simulink model "PTC_MBDS_DeadBand_Sample"  (R2013a)
settings: Solver=FixedStepDiscrete  StartTime=0.0  StopTime=100  FixedStep=Auto  RelTol=1e-3
undefined symbols (not defined in the file): sigbuilder_block
libraries: simulink_extras x1, PTC_MBDS_LIB x1
settings Model: Creator=uidl7367  LastModifiedBy=sundeep.tuteja
settings DataIOCC: SignalLoggingSaveFormat=ModelDataLogs
settings OptimizationCC: ExpressionDepthLimit=2147483647  InitFltsAndDblsToZero=on
settings DebuggingCC: SaveWithParameterizedLinksMsg=none  SignalResolutionControl=TryResolveAllWithWarning  SolverPrmCheckMsg=none  InheritedTsInSrcMsg=none  MultiTaskDSMMsg=warning  MultiTaskCondExecSysMsg=none  FcnCallInpInsideContextMsg=UseLocalSettings  StrictBusMsg=Warning
settings RTWCC: IncludeERTFirstTime=on
settings GRTTargetCC: TargetFcnLib=ansi_tfl_tmw.mat  CombineOutputUpdateFcns=off  GRTInterface=on

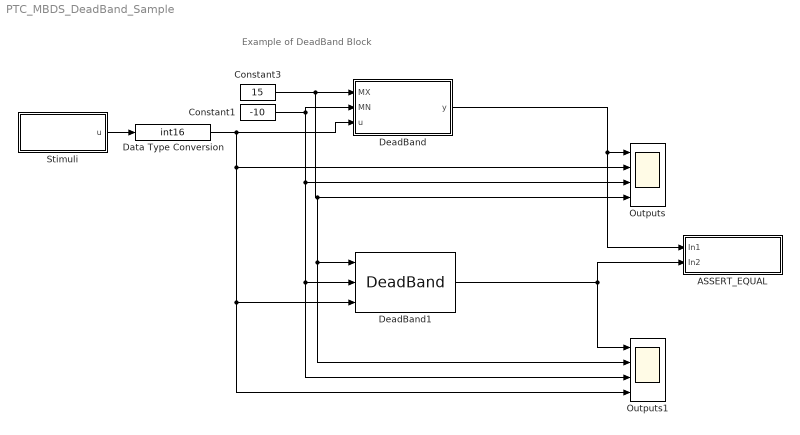
== system PTC_MBDS_DeadBand_Sample ==
  note: Example of DeadBand Block
  ASSERT_EQUAL : Subsystem
  Constant1 : Constant  InitFcn=|  Value=-10  VectorParams1D=off  OutDataTypeStr=Inherit: Inherit via back propagation
      | if(exist('MBDS_BlockCallback', 'file'))
      |    MBDS_BlockCallback('Update', gcb);  
      | end
  Constant3 : Constant  InitFcn=|  Value=15  VectorParams1D=off  OutDataTypeStr=Inherit: Inherit via back propagation
      | if(exist('MBDS_BlockCallback', 'file'))
      |    MBDS_BlockCallback('Update', gcb);  
      | end
  Data Type Conversion : DataTypeConversion  InitFcn=|  OutDataTypeStr=int16  SaturateOnIntegerOverflow=on
      | try
      |    MBDS_BlockCallback('Update', gcb);
      | end
  DeadBand : Subsystem  InitFcn=|  mask(DeadBand){MBDS_LibraryBlock=on, MBDS_BlockVersion=05.40}
      | if(exist('MBDS_BlockCallback', 'file'))
      |    MBDS_BlockCallback('Update', gcb);
      | end
      mask prompts: MBDS_LibraryBlock "MBDS library block"; MBDS_BlockVersion "Block version:"
      mask help: Returns zero, if the input value is between minimum (MN) and maximum (MX). Otherwise the output signal equals to the input signal reduced by the limits.
      mask init:
      | if(exist('MBDS_BlockCallback', 'file'))
      |    MBDS_BlockCallback('Init', gcb);
      | else
      |    % Disable all mask parameters
      |    MaskEnables = get_param(gcb, 'MaskEnables');
      |    for k = [1:length(MaskEnables)]
      |       MaskEnables{k} = 'off';
      |    end
      |    if(~isequal(MaskEnables, get_param(gcb, 'MaskEnables')))
      |       set_param(gcb, 'MaskEnables', MaskEnables);
      |    end
      | end
      mask Help: eval(['open([workdir(''library_dir:''),''\Blockset\help\'',get_param(gcb,''MaskType''),''.html''])'])
      mask Display:
      | % Show icon or block text
      | if(exist('DeadBand.tif', 'file'))
      |    image(imread('DeadBand.tif','tif'), [0.295739348370927 0.17 0.378947368421053 0.66]);
      |    disp('')
      | else
      |    disp(sprintf('Dead\nBand'));
      | end
      | 
      | % Display port labels
      | port_label('input', 1, 'MX');
      | port_label('input', 2, 'MN');
      | port_label('input', 3, 'u');
      | port_label('output', 1, 'y');
  DeadBand1 : PTC_MBDS_LIB/MBDS Standard Library/Basic Operations/Non-Linear Operations/DeadBand  PTC_MBDS_BlockVersion=5.32  PTC_BlockType=PTC_MBDS_DeadBand
  Outputs : Scope  NumInputPorts=4
      settings: TimeRange=10  YMin=-10~-20~-11~14  YMax=0~-10~-9~16  SampleInput=on  SampleTime=1
  Outputs1 : Scope  NumInputPorts=4
      settings: TimeRange=10  YMin=-10~-20~-11~14  YMax=0~-10~-9~16  SampleInput=on  SampleTime=1
  Stimuli : Subsystem  Tag=STV Subsys  LoadFcn=sigbuilder_block('load');  StartFcn=sigbuilder_block('start');  StopFcn=sigbuilder_block('stop');  ClipboardFcn=sigbuilder_block('clipboard');  mask(Sigbuilder block){}
      mask help: Sigbuilder GUI
      mask init:
      | if ~strcmp(get_param(bdroot(gcb),'SimulationStatus'),'stopped') tuvar = sigbuilder_block('maskInit'); end
      settings: CopyFcn=sigbuilder_block('copy');  DeleteFcn=sigbuilder_block('delete');  ModelCloseFcn=sigbuilder_block('modelClose');  PreSaveFcn=sigbuilder_block('preSave');  PauseFcn=sigbuilder_block('pause')  ContinueFcn=sigbuilder_block('continue')  NameChangeFcn=sigbuilder_block('namechange');  OpenFcn=sigbuilder_block('open',[45 129.75 470.25 423.75 ]);  CloseFcn=sigbuilder_block('close');
      mask Display: plot(0,0,100,100,[10,10,40,40,10],[80,20,20,80,80],[40,10],[50,50], [40,27,10],[65,72,56],[40,25,25,10],[28,28,43,43]);
  wires:
  Stimuli/1(u) -> Data Type Conversion/1
  DeadBand/1(y) -> ASSERT_EQUAL/1(In1), Outputs/1
  Constant3/1 -> DeadBand/1(MX), DeadBand1/1, Outputs1/2, Outputs/4
  Constant1/1 -> DeadBand/2(MN), DeadBand1/2, Outputs1/3, Outputs/3
  Data Type Conversion/1 -> DeadBand/3(u), DeadBand1/3, Outputs1/4, Outputs/2
  DeadBand1/1 -> ASSERT_EQUAL/2(In2), Outputs1/1

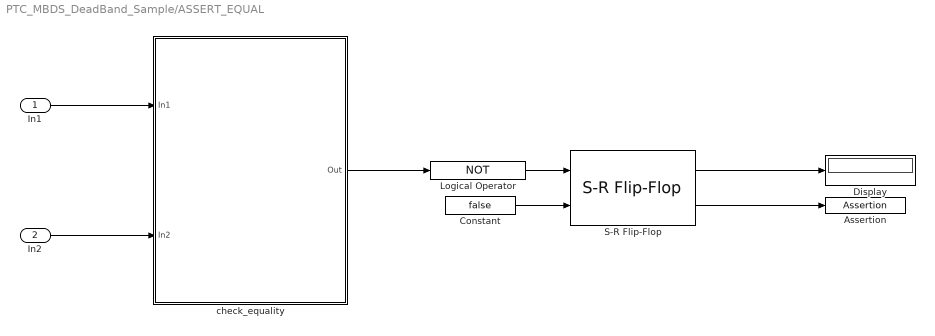
== system PTC_MBDS_DeadBand_Sample/ASSERT_EQUAL ==
  In1 : Inport
  In2 : Inport  Port=2
  Assertion : Assertion
  Constant : Constant  Value=false
  Display : Display
  Logical Operator : Logic  Operator=NOT  AllPortsSameDT=off  OutDataTypeStr=boolean
  S-R Flip-Flop : simulink_extras/Flip Flops/S-R Flip-Flop  initial_condition=0
  check_equality : MATLAB Function  TreatAsAtomicUnit=on
  wires:
  S-R Flip-Flop/1 -> Display/1
  check_equality/1(Out) -> Logical Operator/1
  Constant/1 -> S-R Flip-Flop/2
  S-R Flip-Flop/2 -> Assertion/1
  In2/1 -> check_equality/2(In2)
  In1/1 -> check_equality/1(In1)
  Logical Operator/1 -> S-R Flip-Flop/1

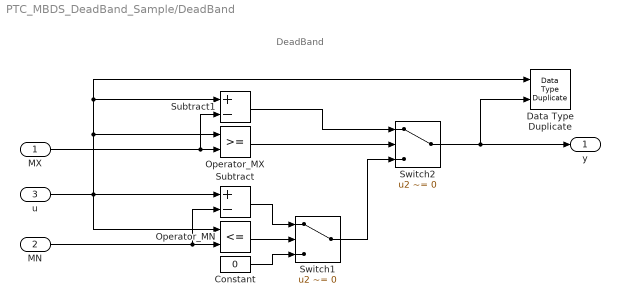
== system PTC_MBDS_DeadBand_Sample/DeadBand ==
  note: DeadBand
  MX : Inport
  MN : Inport  Port=2
  u : Inport  Port=3
  Constant : Constant  Value=0  OutDataTypeStr=Inherit: Inherit via back propagation
  Data Type Duplicate : DataTypeDuplicate
  Operator_MN : RelationalOperator  Operator=<=  OutDataTypeStr=boolean
  Operator_MX : RelationalOperator  OutDataTypeStr=boolean
  Subtract : Sum  Inputs=+-  OutDataTypeStr=Inherit: Inherit via back propagation  SaturateOnIntegerOverflow=on
  Subtract1 : Sum  Inputs=+-  OutDataTypeStr=Inherit: Inherit via back propagation  SaturateOnIntegerOverflow=on
  Switch1 : Switch  Criteria=u2 ~= 0  OutDataTypeStr=Inherit: Inherit via back propagation  SaturateOnIntegerOverflow=on
  Switch2 : Switch  Criteria=u2 ~= 0  OutDataTypeStr=Inherit: Inherit via back propagation  SaturateOnIntegerOverflow=on
  y : Outport
  wires:
  Subtract1/1 -> Switch2/1
  u/1 -> Operator_MX/1, Data Type Duplicate/1, Subtract1/1, Operator_MN/1, Subtract/1
  Constant/1 -> Switch1/3
  Subtract/1 -> Switch1/1
  MN/1 -> Operator_MN/2, Subtract/2
  Switch1/1 -> Switch2/3
  MX/1 -> Operator_MX/2, Subtract1/2
  Operator_MX/1 -> Switch2/2
  Operator_MN/1 -> Switch1/2
  Switch2/1 -> y/1, Data Type Duplicate/2

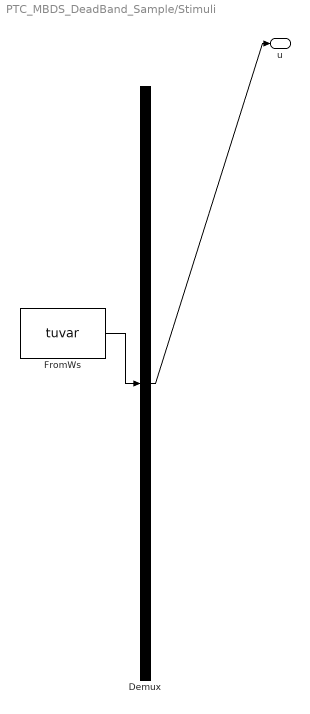
== system PTC_MBDS_DeadBand_Sample/Stimuli ==
  Demux : Demux  Tag=STV Demux  Outputs=1
  FromWs : FromWorkspace  Tag=STV FromWs  VariableName=tuvar  SampleTime=1  OutputAfterFinalValue=Holding final value
      SigBuilderData=|
      | common.afterFinalStr = 'Hold final value'
      | common.sampleTime = 1
      | dataSet.timeRange = [0 10]
      | dataSet.name = 'test data'
      | sbobj.Groups.Name = 'test data'
      | sbobj.Groups.Signals.Name = 'u'
      | sbobj.Groups.Signals.XData = [0 2 4 6 8 10]
      | sbobj.Groups.Signals.YData = [-20 -18 -16 -14 -12 -10]
  u : Outport  Tag=STV Outport
  wires:
  Demux/1 -> u/1
  FromWs/1 -> Demux/1

== matlab function PTC_MBDS_DeadBand_Sample/ASSERT_EQUAL/check_equality ==
  data: In1 input; Out output; In2 input
function Out = check_equality(In1, In2)
%#codegen

Out = isequaln(In1, In2);

end
